simulink model "GravityTanks"  (R2014b)
settings: Solver=ode45  StartTime=0.0  StopTime=20  MaxStep=0.1  RelTol=1e-3
settings Model: Creator=jeff  LastModifiedBy=jeff

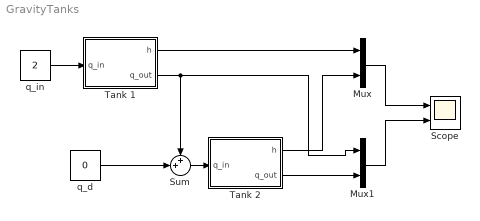
== system GravityTanks ==
  Mux : Mux  Inputs=2
  Mux1 : Mux  Inputs=2
  Scope : Scope  NumInputPorts=2
      settings: TimeRange=20  YMin=0~0  YMax=1.8~2
  Sum : Sum  Inputs=++|
  Tank 1 : Subsystem
  Tank 2 : Subsystem
  q_d : Constant  Value=0
  q_in : Constant  Value=2
  wires:
  q_in/1 -> Tank 1/1(q_in)
  Tank 1/2(q_out) -> Mux1/1, Sum/1
  Tank 1/1(h) -> Mux/1
  Tank 2/1(h) -> Mux/2
  Tank 2/2(q_out) -> Mux1/2
  Mux/1 -> Scope/1
  Mux1/1 -> Scope/2
  Sum/1 -> Tank 2/1(q_in)
  q_d/1 -> Sum/2

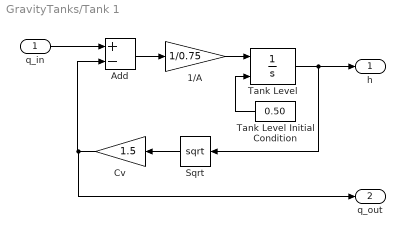
== system GravityTanks/Tank 1 ==
  q_in : Inport
  1/A : Gain  Gain=1/0.75
  Add : Sum  Inputs=+-
  Cv : Gain  Gain=1.5
  Sqrt : Sqrt  SaturateOnIntegerOverflow=on
  Tank Level : Integrator  InitialConditionSource=external  LimitOutput=on  LowerSaturationLimit=0
  Tank Level Initial Condition : Constant  Value=0.50
  h : Outport
  q_out : Outport  Port=2
  wires:
  1/A/1 -> Tank Level/1
  Add/1 -> 1/A/1
  Tank Level/1 -> h/1, Sqrt/1
  Cv/1 -> q_out/1, Add/2
  q_in/1 -> Add/1
  Tank Level Initial Condition/1 -> Tank Level/2
  Sqrt/1 -> Cv/1

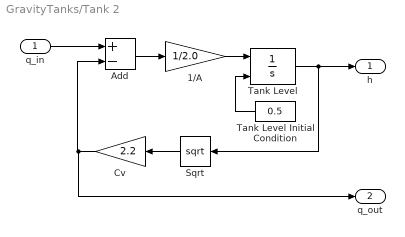
== system GravityTanks/Tank 2 ==
  q_in : Inport
  1/A : Gain  Gain=1/2.0
  Add : Sum  Inputs=+-
  Cv : Gain  Gain=2.2
  Sqrt : Sqrt  SaturateOnIntegerOverflow=on
  Tank Level : Integrator  InitialConditionSource=external  LimitOutput=on  LowerSaturationLimit=0
  Tank Level Initial Condition : Constant  Value=0.5
  h : Outport
  q_out : Outport  Port=2
  wires:
  1/A/1 -> Tank Level/1
  Add/1 -> 1/A/1
  Tank Level/1 -> h/1, Sqrt/1
  Cv/1 -> q_out/1, Add/2
  q_in/1 -> Add/1
  Tank Level Initial Condition/1 -> Tank Level/2
  Sqrt/1 -> Cv/1
